simulink model "Design2RealTime"  (R2024b)
settings: Solver=FixedStepDiscrete  StartTime=0.0  StopTime=10  FixedStep=0.001  RelTol=1e-3
values from neighbouring files (symbols this model uses):
  Ao = F(2, 2) - L * F(1, 2)    [Design1.m]    (also in Design2.m)
  Bo = [G(2) - L * G(1), Ao * L + F(2, 1) - L * F(1, 1)]    [Design1.m]    (also in Design2.m)
  Co = [0; 1]    [Design1.m]    (also in Design2.m)
  Do = [0, 1; 0, L]    [Design1.m]    (also in Design2.m)
  K = place(F, G, DesiredPoles)    [Design1.m]    (also in Design2.m = Ktmp(2:3))
  Nr = Nu + K * Nx    [Design1.m]    (also in Design2.m)
  Ts = TsCand(i)    [Design1.m]    (also in Design2.m)
undefined symbols (not defined in the file or in its folder): DiscIntNeverNeededParam, National_Instruments, PCI, sens
libraries: simulink_extras x3, sldrtlib x2
settings Model: SimulationMode=external  ExtModeTrigDuration=1000001  Creator=galeazzolu  LastModifiedBy=galeazzolu
settings DataIOCC: ReturnWorkspaceOutputs=off
settings HardwareCC: ProdBitPerLong=64  ProdHWDeviceType=Intel->x86-64 (Linux 64)
settings RTWCC: Description=Simulink Desktop Real-Time  SystemTargetFile=sldrt.tlc  TemplateMakefile=sldrt.tmf  RTWCompilerOptimization=on
settings CodeAppCC: MaxIdLength=95
settings SimulinkDesktopRealTimeCC: TargetLibSuffix=_sldrt.a  TargetPreCompLibLocation=C:\Program Files\MATLAB\R2024b\toolbox\sldrt\lib\win64  ParMdlRefBuildCompliant=on

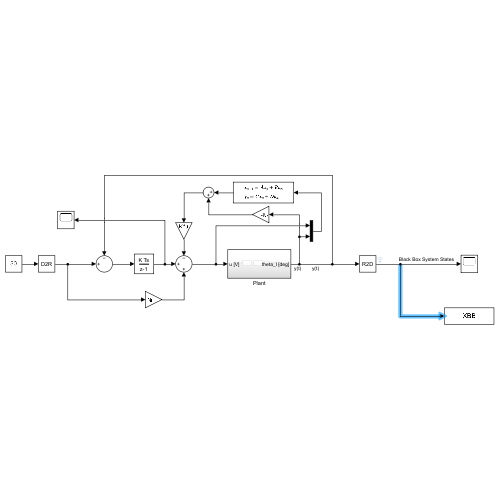
[thumbnail: Simulink's stored preview of the top-level diagram]
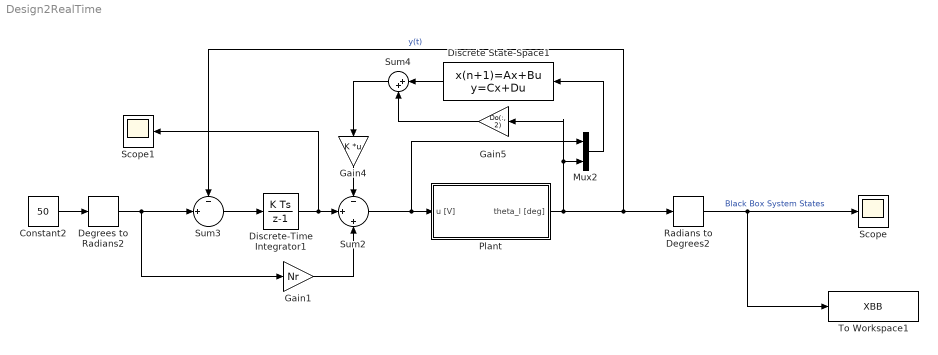
== system Design2RealTime ==
  Constant2 : Constant  Value=50
  Degrees to Radians2 : simulink_extras/Transformations/Degrees to Radians
  Discrete State-Space1 : DiscreteStateSpace  A=Ao  B=Bo  C=Co  D=zeros(2)  SampleTime=Ts
  Discrete-Time Integrator1 : DiscreteIntegrator  gainval=Ki  SampleTime=-1  ICPrevOutput=DiscIntNeverNeededParam  ICPrevScaledInput=DiscIntNeverNeededParam
  Gain1 : Gain  Gain=Nr
  Gain4 : Gain  Gain=K  Multiplication=Matrix(K*u)
  Gain5 : Gain  Gain=Do(:, 2)
  Mux2 : Mux  Inputs=2
  Plant : Subsystem
  Radians to Degrees2 : simulink_extras/Transformations/Radians to Degrees
  Scope : Scope
  Scope1 : Scope
  Sum2 : Sum  Inputs=-|+|+
  Sum3 : Sum  Inputs=-|+||
  Sum4 : Sum  Inputs=|++
  To Workspace1 : ToWorkspace  VariableName=XBB  SaveFormat=Timeseries  SampleTime=-1
  wires:
  Plant/1(theta_l [deg]) -> Sum3/1, Radians to Degrees2/1, Mux2/2, Gain5/1  "y(t)"
  Mux2/1 -> Discrete State-Space1/1
  Sum2/1 -> Mux2/1, Plant/1(u [V])
  Discrete-Time Integrator1/1 -> Scope1/1, Sum2/2
  Constant2/1 -> Degrees to Radians2/1
  Sum3/1 -> Discrete-Time Integrator1/1
  Degrees to Radians2/1 -> Sum3/2, Gain1/1
  Gain1/1 -> Sum2/3
  Discrete State-Space1/1 -> Sum4/1
  Gain4/1 -> Sum2/1
  Sum4/1 -> Gain4/1
  Gain5/1 -> Sum4/2
  Radians to Degrees2/1 -> To Workspace1/1, Scope/1  "Black Box System States"

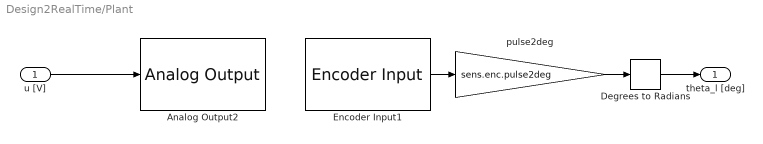
== system Design2RealTime/Plant ==
  u [V] : Inport
  Analog Output2 : sldrtlib/Analog Output  SampleTime=Ts  MaxMissedTicks=10  ShowMissedTicks=off  YieldWhenWaiting=off  DrvName=National_Instruments/PCI-6221  DrvAddress=4294967295  DrvOptions=[0 0 0 2 0]  Channels=1  RangeMode=1  VoltRange=1  InitialValue=0  FinalValue=0
      settings: AttributesFormatString=National Instruments\nPCI-6221 [auto]
  Degrees to Radians : simulink_extras/Transformations/Degrees to Radians
  Encoder Input1 : sldrtlib/Encoder Input  SampleTime=Ts  MaxMissedTicks=10  ShowMissedTicks=off  YieldWhenWaiting=off  DrvName=National_Instruments/PCI-6221  DrvAddress=4294967295  DrvOptions=[0 0 0 2 0]  Channels=1  QuadMode=3  IndexPulse=1  InputFilter=Inf  DataType=1
      settings: AttributesFormatString=National Instruments\nPCI-6221 [auto]
  pulse2deg : Gain  Gain=sens.enc.pulse2deg
  theta_l [deg] : Outport
  wires:
  u [V]/1 -> Analog Output2/1
  Degrees to Radians/1 -> theta_l [deg]/1
  pulse2deg/1 -> Degrees to Radians/1
  Encoder Input1/1 -> pulse2deg/1
